simulink model "foc"  (R2021b)
settings: Solver=FixedStepDiscrete  StartTime=0.0  StopTime=1  FixedStep=1/12000  RelTol=1e-3
libraries: simulink x1
settings Model: Creator=yangqingyao  LastModifiedBy=yangqingyao
settings DebuggingCC: UnconnectedInputMsg=none  UnconnectedOutputMsg=none  UnconnectedLineMsg=none
settings ModelReferenceCC: EnableRefExpFcnMdlSchedulingChecks=off
settings RTWCC: DLArmComputeVersion=20.02.1

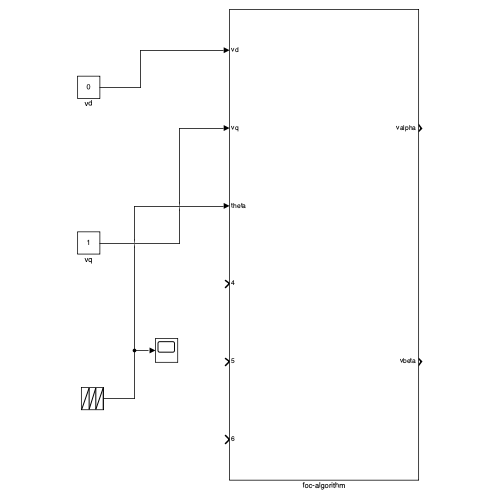
[thumbnail: Simulink's stored preview of the top-level diagram]
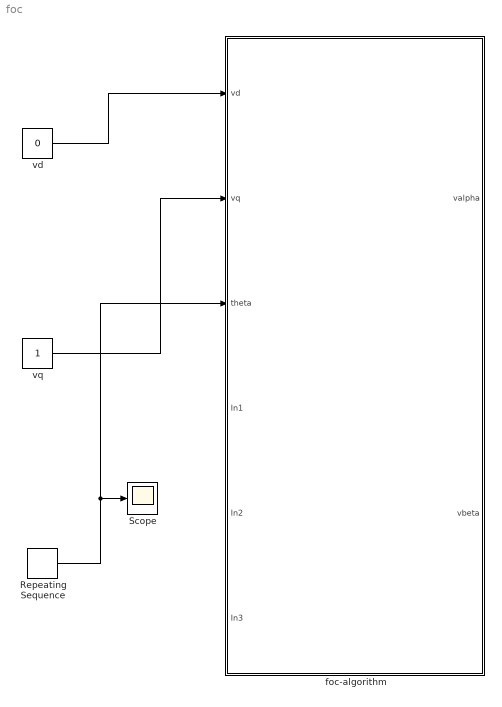
== system foc ==
  Repeating Sequence : simulink/Sources/Repeating Sequence  rep_seq_t=[0,0.1]  rep_seq_y=[0,2*pi]
  Scope : Scope
  foc-algorithm : Subsystem
  vd : Constant  Value=0
  vq : Constant
  wires:
  vd/1 -> foc-algorithm/1(vd)
  vq/1 -> foc-algorithm/2(vq)
  Repeating Sequence/1 -> Scope/1, foc-algorithm/3(theta)

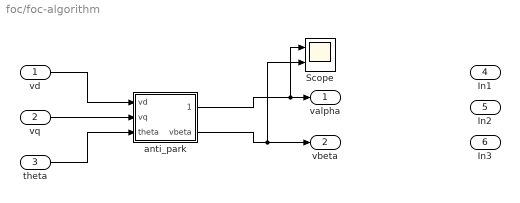
== system foc/foc-algorithm ==
  vd : Inport
  vq : Inport  Port=2
  theta : Inport  Port=3
  In1 : Inport  Port=4
  In2 : Inport  Port=5
  In3 : Inport  Port=6
  Scope : Scope  NumInputPorts=2
  anti_park : Subsystem
  valpha : Outport
  vbeta : Outport  Port=2
  wires:
  vd/1 -> anti_park/1(vd)
  vq/1 -> anti_park/2(vq)
  theta/1 -> anti_park/3(theta)
  anti_park/1(valpha) -> Scope/1, valpha/1
  anti_park/2(vbeta) -> Scope/2, vbeta/1

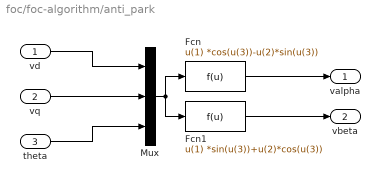
== system foc/foc-algorithm/anti_park ==
  vd : Inport
  vq : Inport  Port=2
  theta : Inport  Port=3
  Fcn : Fcn  Expr=u(1) *cos(u(3))-u(2)*sin(u(3))
  Fcn1 : Fcn  Expr=u(1) *sin(u(3))+u(2)*cos(u(3))
  Mux : Mux  Inputs=3
  valpha : Outport
  vbeta : Outport  Port=2
  wires:
  vq/1 -> Mux/2
  vd/1 -> Mux/1
  Fcn/1 -> valpha/1
  Mux/1 -> Fcn1/1, Fcn/1
  theta/1 -> Mux/3
  Fcn1/1 -> vbeta/1
